simulink model "plant"  (R2025b)
settings: Solver=FixedStepAuto  StartTime=0.0  StopTime=10.0  RelTol=1e-3
undefined symbols (not defined in the file): g, Gamma, J, J_inv, m, rotors_max, rotors_min, tau_m
libraries: matrix_library x1
settings Model: DataDictionary=project.sldd  Creator=Nick  LastModifiedBy=Nick

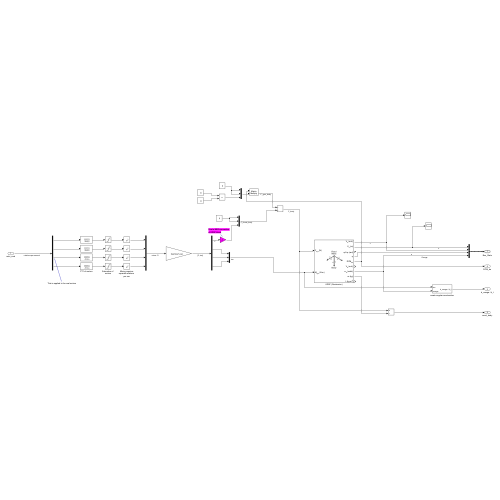
[thumbnail: Simulink's stored preview of the top-level diagram]
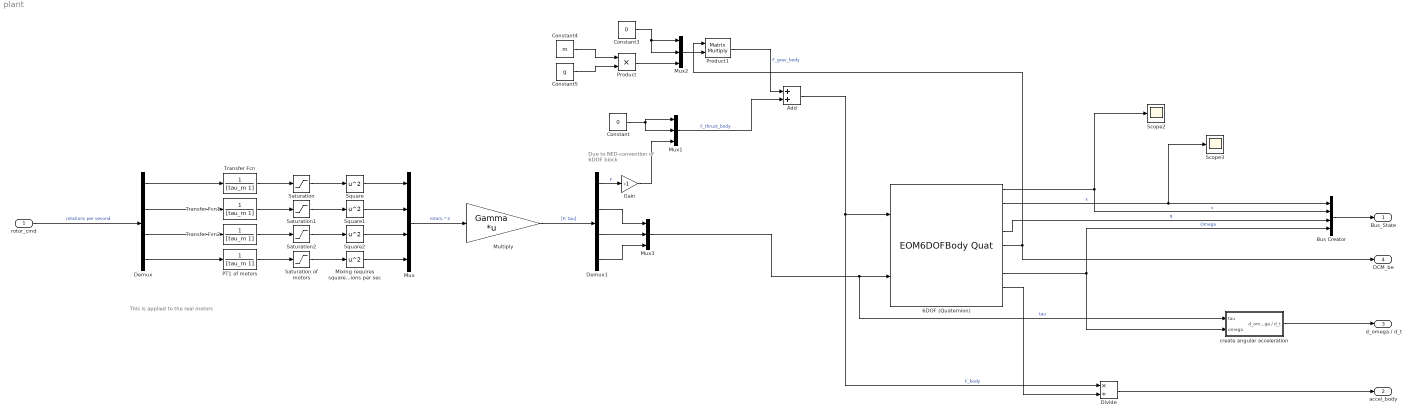
== system plant ==
  note: This is applied to the real motors
  note: Due to NED-convention
      | of 6DOF block
  rotor_cmd : Inport
  6DOF (Quaternion) : EOM6DOFBodyQuat  mass_0=m  inertia=J  mass_flag=on
  Add : Sum
  Bus Creator : BusCreator  Inputs=4  OutDataTypeStr=Bus: Bus_State  NonVirtualBus=on
  Constant : Constant  Value=0
  Constant3 : Constant  Value=0
  Constant4 : Constant  Value=m
  Constant5 : Constant  Value=g
  Demux : Demux
  Demux1 : Demux
  Divide : Product  Inputs=*/
  Gain : Gain  Gain=-1
  Mixing requires squared rotations per sec : Math  Operator=square
  Multiply : Gain  Gain=Gamma  Multiplication=Matrix(K*u) (u vector)
  Mux : Mux
  Mux1 : Mux  Inputs=3
  Mux2 : Mux  Inputs=3
  Mux3 : Mux  Inputs=3
  PT1 of motors : TransferFcn  Denominator=[tau_m 1]
  Product : Product
  Product1 : Product  Multiplication=Matrix(*)
  Saturation : Saturate  UpperLimit=rotors_max  LowerLimit=rotors_min
  Saturation of motors : Saturate  UpperLimit=rotors_max  LowerLimit=rotors_min
  Saturation1 : Saturate  UpperLimit=rotors_max  LowerLimit=rotors_min
  Saturation2 : Saturate  UpperLimit=rotors_max  LowerLimit=rotors_min
  Scope2 : Scope
      settings: ActiveDisplayYMinimum=-1  ActiveDisplayYMaximum=1  DataLoggingVariableName=ScopeData2
  Scope3 : Scope
      settings: ActiveDisplayYMinimum=-0.29618772596467313  ActiveDisplayYMaximum=1.1469685459844743  DataLoggingVariableName=ScopeData3
  Square : Math  Operator=square
  Square1 : Math  Operator=square
  Square2 : Math  Operator=square
  Transfer Fcn : TransferFcn  Denominator=[tau_m 1]
  Transfer Fcn1 : TransferFcn  Denominator=[tau_m 1]
  Transfer Fcn2 : TransferFcn  Denominator=[tau_m 1]
  create angular acceleration : Subsystem
  Bus_State : Outport  OutDataTypeStr=Bus: Bus_State
  accel_body : Outport  Port=2
  d_omega / d_t : Outport  Port=3
  DCM_be : Outport  Port=4
  wires:
  Transfer Fcn/1 -> Saturation/1
  Bus Creator/1 -> Bus_State/1
  Demux/1 -> Transfer Fcn/1
  Transfer Fcn1/1 -> Saturation1/1
  Demux/2 -> Transfer Fcn1/1
  Transfer Fcn2/1 -> Saturation2/1
  Demux/3 -> Transfer Fcn2/1
  PT1 of motors/1 -> Saturation of motors/1
  Demux/4 -> PT1 of motors/1
  Saturation/1 -> Square/1
  Saturation1/1 -> Square1/1
  Saturation2/1 -> Square2/1
  Square2/1 -> Mux/3
  Square1/1 -> Mux/2
  Square/1 -> Mux/1
  Mux/1 -> Multiply/1  "rotors.^2"
  Multiply/1 -> Demux1/1  "[F; tau]"
  Constant/1 -> Mux1/1, Mux1/2
  Demux1/1 -> Gain/1  "F"
  Gain/1 -> Mux1/3
  Constant3/1 -> Mux2/1, Mux2/2
  Product/1 -> Mux2/3
  Constant4/1 -> Product/1
  Constant5/1 -> Product/2
  Mux2/1 -> Product1/2
  6DOF (Quaternion)/5 -> DCM_be/1, Product1/1
  Product1/1 -> Add/1  "F_grav_body"
  Mux1/1 -> Add/2  "F_thrust_body"
  Add/1 -> Divide/1, 6DOF (Quaternion)/1  "F_body"
  Mux3/1 -> create angular acceleration/1(tau), 6DOF (Quaternion)/2  "tau"
  Demux1/3 -> Mux3/2
  Demux1/2 -> Mux3/1
  Demux1/4 -> Mux3/3
  6DOF (Quaternion)/7 -> create angular acceleration/2(omega), Bus Creator/4  "Omega"
  6DOF (Quaternion)/2 -> Bus Creator/1, Scope3/1  "x"
  6DOF (Quaternion)/1 -> Scope2/1, Bus Creator/2  "v"
  6DOF (Quaternion)/4 -> Bus Creator/3  "q"
  Divide/1 -> accel_body/1
  create angular acceleration/1(d_omega / d_t) -> d_omega / d_t/1
  rotor_cmd/1 -> Demux/1  "rotations per second"
  6DOF (Quaternion)/8 -> Divide/2
  Mixing requires squared rotations per sec/1 -> Mux/4
  Saturation of motors/1 -> Mixing requires squared rotations per sec/1

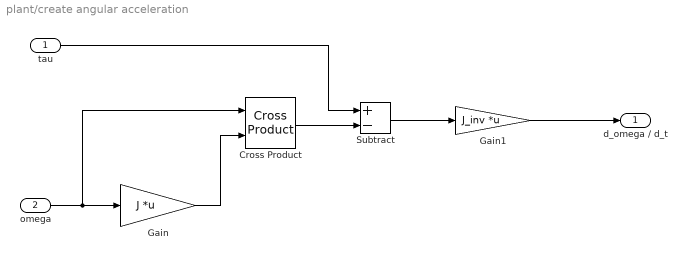
== system plant/create angular acceleration ==
  tau : Inport
  omega : Inport  Port=2
  Cross Product : matrix_library/Cross Product
  Gain : Gain  Gain=J  Multiplication=Matrix(K*u) (u vector)
  Gain1 : Gain  Gain=J_inv  Multiplication=Matrix(K*u) (u vector)
  Subtract : Sum  Inputs=+-
  d_omega / d_t : Outport
  wires:
  omega/1 -> Cross Product/1, Gain/1
  Gain/1 -> Cross Product/2
  Cross Product/1 -> Subtract/2
  tau/1 -> Subtract/1
  Subtract/1 -> Gain1/1
  Gain1/1 -> d_omega / d_t/1
